simulink model "pv_storage_system"  (R2026a)
settings: Solver=ode23tb
values from neighbouring files (symbols this model uses):
  Batt_AhRated = 100    [pv_storage_params.m]
  f_sw_bb = 8e3    (= 8000)    [pv_storage_params.m]
  f_sw_boost = 8e3    (= 8000)    [pv_storage_params.m]
  R1_boost = 0.01    [pv_storage_params.m]
  R_snubber = 2.7    [pv_storage_params.m]
  R_test_load = 480^2 / 30000    (= 7.68)    [pv_storage_params.m]
  R_test_load_batt = 500    [pv_storage_params.m]
  Ts_control = 150e-6    (= 0.00015)    [pv_storage_params.m]
libraries: fl_lib x19, nesl_utility x9, ee_lib x4, ee_lib_for_power_systems x3, simulink x3, batteryecm_lib x1, slpidlib x1
settings Model: Creator=inspiredkhalid  LastModifiedBy=inspiredkhalid

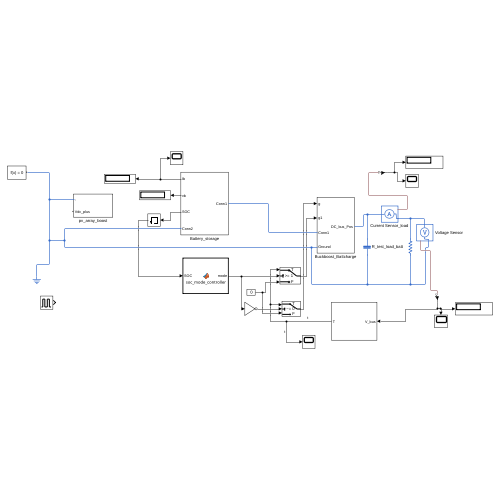
[thumbnail: Simulink's stored preview of the top-level diagram]
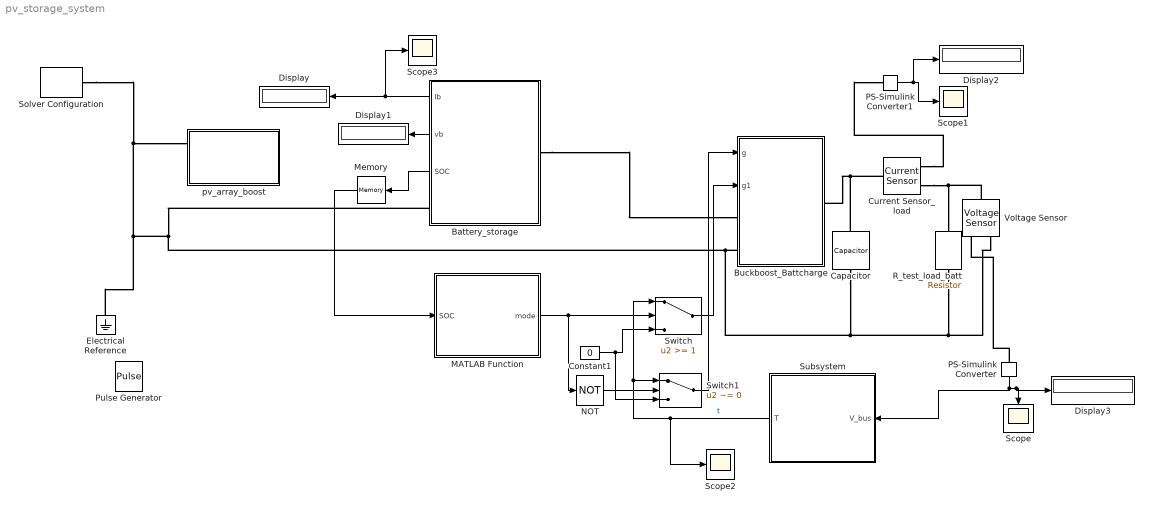
== system pv_storage_system ==
  Battery_storage : Subsystem
  Buckboost_Battcharge : Subsystem
  Capacitor : fl_lib/Electrical/Electrical Elements/Capacitor  c=Cdc F  r=1e-6 Ohm  g=0 1/Ohm  i_specify=off  i_priority=None  i=0 A  i_nominal_specify=off  i_nominal_value=1  i_nominal_unit=A  v_specify=off  v_priority=None  v=0 V  v_nominal_specify=off  v_nominal_value=1  v_nominal_unit=V  vc_specify=off  vc_priority=High  vc=0 V  vc_nominal_specify=off  vc_nominal_value=1  vc_nominal_unit=V
  Constant1 : Constant  Value=0
  Current Sensor_load : fl_lib/Electrical/Electrical Sensors/Current Sensor
  Display{,1..3} (4 alike) : Display
  Electrical Reference : fl_lib/Electrical/Electrical Elements/Electrical Reference
  MATLAB Function : MATLAB Function  TreatAsAtomicUnit=on
  Memory : Memory
  NOT : Logic  Operator=NOT  IconShape=distinctive  AllPortsSameDT=off  OutDataTypeStr=boolean
  PS-Simulink Converter : nesl_utility/PS-Simulink Converter  PhysicalDomain=network_engine_domain  SubClassName=ps_output  LeftPortType=input  RightPortType=output  PseudoPeriodic=off  Frequencies=[]  VectorFormat=inherit  Unit=inherit  AffineConversion=off
  PS-Simulink Converter1 : nesl_utility/PS-Simulink Converter  PhysicalDomain=network_engine_domain  SubClassName=ps_output  LeftPortType=input  RightPortType=output  PseudoPeriodic=off  Frequencies=[]  VectorFormat=inherit  Unit=inherit  AffineConversion=off
  Pulse Generator : DiscretePulseGenerator  PulseType=Time based  Period=1/f_sw_bb  PulseWidth=5
  R_test_load_batt : fl_lib/Electrical/Electrical Elements/Resistor  R=R_test_load_batt Ohm  i_specify=off  i_priority=None  i=0 A  i_nominal_specify=off  i_nominal_value=1  i_nominal_unit=A  v_specify=off  v_priority=None  v=0 V  v_nominal_specify=off  v_nominal_value=1  v_nominal_unit=V
  Scope{,1..3} (4 alike) : Scope
      Scope settings: ActiveDisplayYMinimum=-510.77769359361685  ActiveDisplayYMaximum=637.473510774474  DataLoggingVariableName=ScopeData5
      Scope1 settings: DataLoggingVariableName=ScopeData6
      Scope2 settings: ActiveDisplayYMinimum=0.44778568340914426  ActiveDisplayYMaximum=0.45061540552074841  DataLoggingVariableName=ScopeData7
      Scope3 settings: DataLoggingVariableName=ScopeData9
  Solver Configuration : nesl_utility/Solver Configuration  PhysicalDomain=network_engine_domain  SubClassName=solver  LeftPortType=input  RightPortType=generic  Tones=[]  Harmonics=[]  SimulateNoise=off  Profile=off  UseLocalSampling=off  EnableSwitchedLinearOptims=on  FrequencyDomain=off  UseCCode=off  RelTol=0.001  AbsTol=0.001  MinStep=1e-09  ToWorkspace=off  RevertToSquareIcSolve=off  NumHomotopyIterations=100  PhasorMode=off  PhasorModeNumHarmonics=1  ConsistencySolver=NEWTON_XTOL_AFTER_FTOL  CanonicalOrdering=CANONICAL  OptimizeIntermediates=OPTIMIZED  IndexReductionMethod=DerivativeReplacement  DoDC=off  ResidualTolerance=1e-09  ConsistencyTolSource=GLOBAL  ConsistencyAbsTol=0.001  ConsistencyRelTol=0.001  ConsistencyTolFactor=0.001  UseLocalSolver=on  LocalSolverChoice=NE_TRAPEZOIDAL_ADVANCER  ResolveIndetEquations=on  FunctionEvalNumThread=1  LocalSolverSampleTime=Ts_power  DoFixedCost=off  MaxNonlinIter=3  MaxModeIter=2  ComputeImpulses=off  ImpulseIterations=2  LinearAlgebra=auto  LinearAlgebraNumThread=0  EquationFormulation=NE_TIME_EF  DelaysMemoryBudget=1024  AutomaticFiltering=on  FilteringTimeConstant=0.001  PartitionStorageMethod=AS_NEEDED  PartitionMemoryBudget=1024  PartitionMethod=ROBUST  MultibodyUseLocalSolver=off  MultibodyLocalSolverChoice=ODE1  MultibodyLocalSolverSampleTime=0.001
  Subsystem : Subsystem
  Switch : Switch  Threshold=1  SaturateOnIntegerOverflow=off  InputSameDT=off
  Switch1 : Switch  Criteria=u2 ~= 0  Threshold=1  SaturateOnIntegerOverflow=off  InputSameDT=off
  "Voltage Sensor " : fl_lib/Electrical/Electrical Sensors/Voltage Sensor
  pv_array_boost : Subsystem
  wires:
  Battery_storage/1(Ib) -> Scope3/1, Display/1
  Battery_storage/2(vb) -> Display1/1
  MATLAB Function/1(mode) -> NOT/1, Switch/2
  Subsystem/1(T) -> Scope2/1, Switch/1, Switch1/1  "t"
  Constant1/1 -> Switch1/3, Switch/3
  NOT/1 -> Switch1/2
  Battery_storage/3(SOC) -> Memory/1
  Memory/1 -> MATLAB Function/1(SOC)
  PS-Simulink Converter/1 -> Display3/1, Scope/1, Subsystem/1(V_bus)
  PS-Simulink Converter1/1 -> Display2/1, Scope1/1
  Switch/1 -> Buckboost_Battcharge/2(g1)
  Switch1/1 -> Buckboost_Battcharge/1(g)
  connections:
  Battery_storage/RConn1 -- "Voltage Sensor "/RConn2 -- R_test_load_batt/RConn1 -- Capacitor/RConn1 -- Buckboost_Battcharge/LConn2 -- Electrical Reference/LConn1 -- Solver Configuration/RConn1 -- pv_array_boost/LConn1
  Battery_storage/LConn1 -- Buckboost_Battcharge/LConn1
  "Voltage Sensor "/LConn1 -- Current Sensor_load/RConn2 -- R_test_load_batt/LConn1
  PS-Simulink Converter/LConn1 -- "Voltage Sensor "/RConn1
  Current Sensor_load/LConn1 -- Capacitor/LConn1 -- Buckboost_Battcharge/RConn1
  Current Sensor_load/RConn1 -- PS-Simulink Converter1/LConn1

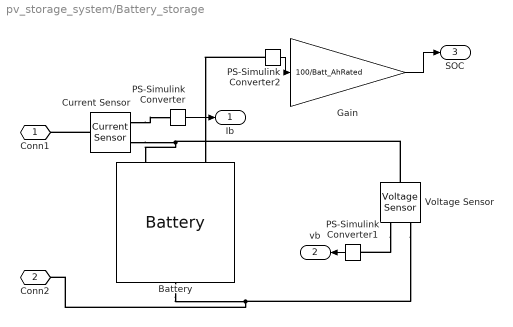
== system pv_storage_system/Battery_storage ==
  Battery : batteryecm_lib/Battery  Vnom=Batt_Vnom V  prm_dir=simscape.enum.battery.prm_dir.disabled  R1_dis=2 Ohm  R1_ch=2 Ohm  R1=Batt_Rint Ohm  prm_AH=simscape.enum.battery.prm_AH.finite  AH=Batt_AhRated A*hr  V1=Batt_V1_calib V  AH1=Batt_AH1_calib A*hr  prm_R2=simscape.enum.battery.prm_R2.disabled  R2=2000 Ohm  Tmeas=298.15 K  charge_measurement_port=simscape.enum.battery.enable.yes  prm_dyn=simscape.enum.battery.prm_dyn.off  Rp1=0.005 Ohm  tau1=30 s  Rp2=0.005 Ohm  tau2=30 s  Rp3=0.005 Ohm  tau3=30 s  Rp4=0.005 Ohm  tau4=30 s  Rp5=0.005 Ohm  tau5=30 s  prm_fade=simscape.enum.battery.prm_fade.disabled  N_fade=100  AH_fade=45 A*hr  R1_fade=2.02 Ohm  R1_ch_fade=2.02 Ohm  V1_fade=10.35 V  prm_age=simscape.enum.battery.prm_age.disabled  prm_age_OCV=simscape.enum.battery.prm_age_OCV.OCV  OCV_age=0.9  SOC_age=60  Tmeas_age=298.15 K  delta_time_age_vec=[0] d  temperature_age_vec=[273] K  OCV_scaling_age=2.2134e6  OCV_offset_age=1.632e6  temp_exp_age=0.515833569 V  t_exp_age=0.75  Vnom_T2=12 V  R1_T2=2.2 Ohm  R1_T2_dis=2.2 Ohm  R1_T2_ch=2.2 Ohm  V1_T2=11.4 V  R2_T2=2200 Ohm  Rp1_T2=0.005 Ohm  tau1_T2=30 s  Rp2_T2=0.005 Ohm  tau2_T2=30 s  Rp3_T2=0.005 Ohm  tau3_T2=30 s  Rp4_T2=0.005 Ohm  tau4_T2=30 s  Rp5_T2=0.005 Ohm  tau5_T2=30 s  Tmeas2=273.15 K  thermal_port=simscape.enum.thermaleffects.omit  thermal_mass=30000 J/K  i_specify=off  i_priority=None  i=0 A  i_nominal_specify=off  i_nominal_value=1  i_nominal_unit=A  v_specify=off  v_priority=None  v=0 V  v_nominal_specify=off  v_nominal_value=1  v_nominal_unit=V  charge_specify=on  charge_priority=High  charge=Batt_Charge_init A*hr  charge_nominal_specify=off  charge_nominal_value=1  charge_nominal_unit=A*hr  num_cycles_specify=off  num_cycles_priority=High  num_cycles=0  num_cycles_nominal_specify=off  num_cycles_nominal_value=1  num_cycles_nominal_unit=1  temperature_specify=off  temperature_priority=High  temperature=298.15 K  temperature_nominal_specify=off  temperature_nominal_value=1  temperature_nominal_unit=K
  Current Sensor : fl_lib/Electrical/Electrical Sensors/Current Sensor
  Gain : Gain  Gain=100/Batt_AhRated
  PS-Simulink Converter : nesl_utility/PS-Simulink Converter  PhysicalDomain=network_engine_domain  SubClassName=ps_output  LeftPortType=input  RightPortType=output  PseudoPeriodic=off  Frequencies=[]  VectorFormat=inherit  Unit=inherit  AffineConversion=off
  PS-Simulink Converter1 : nesl_utility/PS-Simulink Converter  PhysicalDomain=network_engine_domain  SubClassName=ps_output  LeftPortType=input  RightPortType=output  PseudoPeriodic=off  Frequencies=[]  VectorFormat=inherit  Unit=inherit  AffineConversion=off
  PS-Simulink Converter2 : nesl_utility/PS-Simulink Converter  PhysicalDomain=network_engine_domain  SubClassName=ps_output  LeftPortType=input  RightPortType=output  PseudoPeriodic=off  Frequencies=[]  VectorFormat=inherit  Unit=inherit  AffineConversion=off
  Voltage Sensor : fl_lib/Electrical/Electrical Sensors/Voltage Sensor
  Conn1 : PMIOPort  Side=Left
  Conn2 : PMIOPort  Port=2  Side=Right
  Ib : Outport
  vb : Outport  Port=2
  SOC : Outport  Port=3
  wires:
  PS-Simulink Converter/1 -> Ib/1
  PS-Simulink Converter1/1 -> vb/1
  PS-Simulink Converter2/1 -> Gain/1
  Gain/1 -> SOC/1
  connections:
  Battery/RConn1 -- Voltage Sensor/RConn2 -- Conn2/RConn1
  Current Sensor/LConn1 -- Conn1/RConn1
  Voltage Sensor/LConn1 -- Current Sensor/RConn2 -- Battery/LConn1
  Current Sensor/RConn1 -- PS-Simulink Converter/LConn1
  Voltage Sensor/RConn1 -- PS-Simulink Converter1/LConn1
  PS-Simulink Converter2/LConn1 -- Battery/LConn2

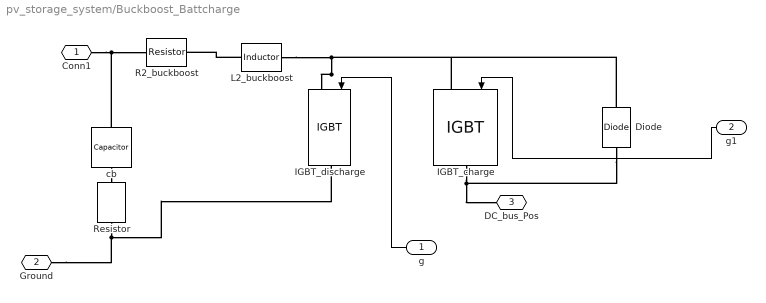
== system pv_storage_system/Buckboost_Battcharge ==
  g : Inport
  g1 : Inport  Port=2
  " IGBT_charge" : ee_lib_for_power_systems/Power Converters/IGBT  Vf=0.6  Ron=1e-3  Goff=1e-5  run_time=off
      settings: SourceProductName=Support Library for Power Systems
  Diode : fl_lib/Electrical/Electrical Elements/Diode  Vf=0.6 V  Ron=0.3 Ohm  Goff=1e-8 1/Ohm  i_specify=off  i_priority=None  i=0 A  i_nominal_specify=off  i_nominal_value=1  i_nominal_unit=A  v_specify=off  v_priority=None  v=0 V  v_nominal_specify=off  v_nominal_value=1  v_nominal_unit=V
  IGBT_discharge : ee_lib_for_power_systems/Power Converters/IGBT  Vf=0.6  Ron=1e-3  Goff=1e-5  run_time=off
      settings: SourceProductName=Support Library for Power Systems
  L2_buckboost : ee_lib/Passive/Inductor  l=1e-6 H  enable_L_tol=ee.enum.toleranceApplication.none  L_tol=20  tol_distribution=ee.enum.toleranceDistribution.uniform  nSigma=4  r=0 Ohm  g=1e-9 1/Ohm  enable_operating_limits=ee.enum.enable.no  operating_limit_action=ee.enum.passive.reportOpLim.warn  max_working_current=1 A  power_rating=1 W  i_L_specify=off  i_L_priority=High  i_L=0 A  i_L_nominal_specify=off  i_L_nominal_value=1  i_L_nominal_unit=A
  R2_buckboost : fl_lib/Electrical/Electrical Elements/Resistor  R=1 Ohm  i_specify=off  i_priority=None  i=0 A  i_nominal_specify=off  i_nominal_value=1  i_nominal_unit=A  v_specify=off  v_priority=None  v=0 V  v_nominal_specify=off  v_nominal_value=1  v_nominal_unit=V
  Resistor : fl_lib/Electrical/Electrical Elements/Resistor  R=R_snubber Ohm  i_specify=off  i_priority=None  i=0 A  i_nominal_specify=off  i_nominal_value=1  i_nominal_unit=A  v_specify=off  v_priority=None  v=0 V  v_nominal_specify=off  v_nominal_value=1  v_nominal_unit=V
  cb : fl_lib/Electrical/Electrical Elements/Capacitor  c=1e-6 F  r=1e-6 Ohm  g=0 1/Ohm  i_specify=off  i_priority=None  i=0 A  i_nominal_specify=off  i_nominal_value=1  i_nominal_unit=A  v_specify=off  v_priority=None  v=0 V  v_nominal_specify=off  v_nominal_value=1  v_nominal_unit=V  vc_specify=off  vc_priority=High  vc=0 V  vc_nominal_specify=off  vc_nominal_value=1  vc_nominal_unit=V
  Conn1 : PMIOPort  Side=Left
  Ground : PMIOPort  Port=2  Side=Left
  DC_bus_Pos : PMIOPort  Port=3  Side=Right
  wires:
  g/1 -> IGBT_discharge/1
  g1/1 -> " IGBT_charge"/1
  connections:
  " IGBT_charge"/RConn1 -- DC_bus_Pos/RConn1 -- Diode/RConn1
  IGBT_discharge/LConn1 -- Diode/LConn1 -- " IGBT_charge"/LConn1 -- L2_buckboost/RConn1
  cb/LConn1 -- R2_buckboost/LConn1 -- Conn1/RConn1
  L2_buckboost/LConn1 -- R2_buckboost/RConn1
  Ground/RConn1 -- IGBT_discharge/RConn1 -- Resistor/RConn1
  cb/RConn1 -- Resistor/LConn1

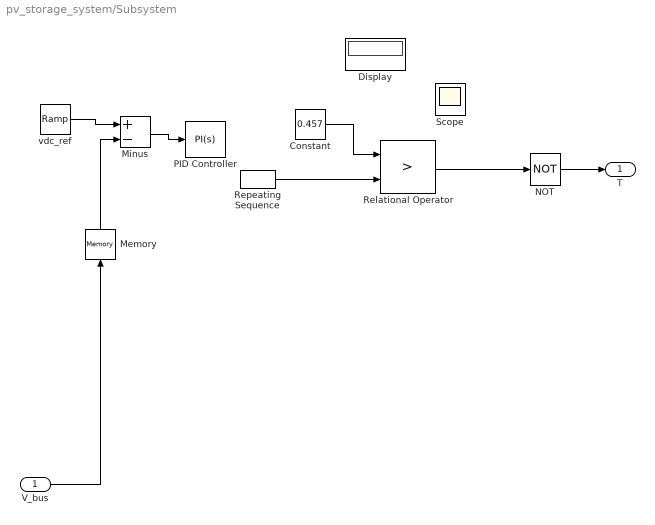
== system pv_storage_system/Subsystem ==
  V_bus : Inport
  Constant : Constant  Value=0.457
  Display : Display
  Memory : Memory
  Minus : Sum  Inputs=+-
  NOT : Logic  Operator=NOT  IconShape=distinctive  AllPortsSameDT=off  OutDataTypeStr=boolean
  PID Controller : slpidlib/PID Controller  Controller=PI  Form=Parallel  TimeDomain=Continuous-time  UseExternalTs=off  SampleTime=-1  IntegratorMethod=Forward Euler  FilterMethod=Forward Euler  ControllerParametersSource=internal  P=0.001  I=0.1  UseKiTs=off  D=0  UseExternalDerivativeSource=off  N=100  UseFilter=on  TunerSelectOption=Transfer Function Based (PID Tuner App)  InitialConditionSource=internal  InitialConditionForIntegrator=0  InitialConditionForFilter=0  DifferentiatorICPrevScaledInput=0  ExternalReset=none  TrackingMode=off  Kt=1  LimitOutput=on  SatLimitsSource=internal  UpperSaturationLimit=0.85  LowerSaturationLimit=0  LinearizeAsGain=on  AntiWindupMode=clamping  Kb=1  LimitIntegrator=off  UpperIntegratorSaturationLimit=inf  LowerIntegratorSaturationLimit=-inf  POutMin=[]  POutMax=[]  IOutMin=[]  IOutMax=[]  DOutMin=[]  DOutMax=[]  NOutMin=[]  NOutMax=[]  SumOutMin=[]  SumOutMax=[]  SaturationOutMin=[]  SaturationOutMax=[]  PParamMin=[]  PParamMax=[]  IParamMin=[]  IParamMax=[]  DParamMin=[]  DParamMax=[]  NParamMin=[]  NParamMax=[]  KbParamMin=[]  KbParamMax=[]  KtParamMin=[]  KtParamMax=[]  KbOutMin=[]  KbOutMax=[]  KtOutMin=[]  KtOutMax=[]  IntegratorOutMin=[]  IntegratorOutMax=[]  FilterOutMin=[]  FilterOutMax=[]  SumI1OutMin=[]  SumI1OutMax=[]  SumI2OutMin=[]  SumI2OutMax=[]  SumI3OutMin=[]  SumI3OutMax=[]  SumI4OutMin=[]  SumI4OutMax=[]  SumDOutMin=[]  SumDOutMax=[]  DifferentiatorOutMin=[]  DifferentiatorOutMax=[]  FilterDiffOutCoefMin=[]  FilterDiffOutCoefMax=[]  ReciprocalOutMin=[]  ReciprocalOutMax=[]  SumDenOutMin=[]  SumDenOutMax=[]  SumNumOutMin=[]  SumNumOutMax=[]  DivideOutMin=[]  DivideOutMax=[]  UdiffTsProdOutMin=[]  UdiffTsProdOutMax=[]  NTsProdOutMin=[]  NTsProdOutMax=[]  UintegralTsProdOutMin=[]  UintegralTsProdOutMax=[]  UngainTsProdOutMin=[]  UngainTsProdOutMax=[]  ClampingZeroOutDataTypeStr=Inherit: Inherit via back propagation  ClampingZeroOutMin=[]  ClampingZeroOutMax=[]  FilterDenConstantOutDataTypeStr=Inherit: Inherit via back propagation  FilterDenConstantOutMin=[]  FilterDenConstantOutMax=[]  PCopyOutDataTypeStr=Inherit: Inherit via back propagation  PCopyOutMin=[]  PCopyOutMax=[]  NCopyOutDataTypeStr=Inherit: Inherit via back propagation  NCopyOutMin=[]  NCopyOutMax=[]  IntegratorContinuousStateAttributes=''  IntegratorStateMustResolveToSignalObject=off  IntegratorRTWStateStorageClass=Auto  FilterContinuousStateAttributes=''  FilterStateMustResolveToSignalObject=off  FilterRTWStateStorageClass=Auto  ParallelPVariant=InternalParameters  IdealPVariant=Disabled  IVariant=InternalParameters  DVariant=Disabled  IntegratorVariant=Continuous  SatVariant=Enabled  AWVariant=ContClampingParallel  PCopyVariant=Disabled  TRVariant=Disabled  FdbkBlocksVariant=Forward  IdealPFdbkVariant=Disabled  SatFdbkVariant=Disabled  DerivativeFilterVariant=Disabled  NVariant=Disabled  NCopyVariant=Disabled_SignalSpec  FilterICVariant=Disabled  IntegratorICVariant=InternalICs  ExternalResetVariant=Disabled  TRSumVariant=Passthrough  SumFdbkVariant=Disabled  SumVariant=Sum_PI  TsampFilterVariant=InternalTs  TsampNgainVariant=Passthrough  TsampIntegralVariant=Disabled_SignalSpec  ExternalSaturationOutDataTypeStr=Inherit: Same as second input  DerivativeSourceVariant=Disabled  PreIntVariant=InternalPreInt
  Relational Operator : RelationalOperator  Operator=>  OutDataTypeStr=boolean  RndMeth=Simplest  InputSameDT=off
  Repeating Sequence : simulink/Sources/Repeating Sequence  rep_seq_t=[0 1/f_sw_bb]  rep_seq_y=[0 1]
  Scope : Scope
      settings: ActiveDisplayYMinimum=0.96541730097571365  ActiveDisplayYMaximum=1.0189869647757612  DataLoggingVariableName=ScopeData8
  vdc_ref : simulink/Sources/Ramp  slope=500  start=0  InitialOutput=0
  T : Outport
  wires:
  Repeating Sequence/1 -> Relational Operator/2
  Minus/1 -> PID Controller/1
  vdc_ref/1 -> Minus/1
  V_bus/1 -> Memory/1
  Memory/1 -> Minus/2
  NOT/1 -> T/1
  Relational Operator/1 -> NOT/1
  Constant/1 -> Relational Operator/1

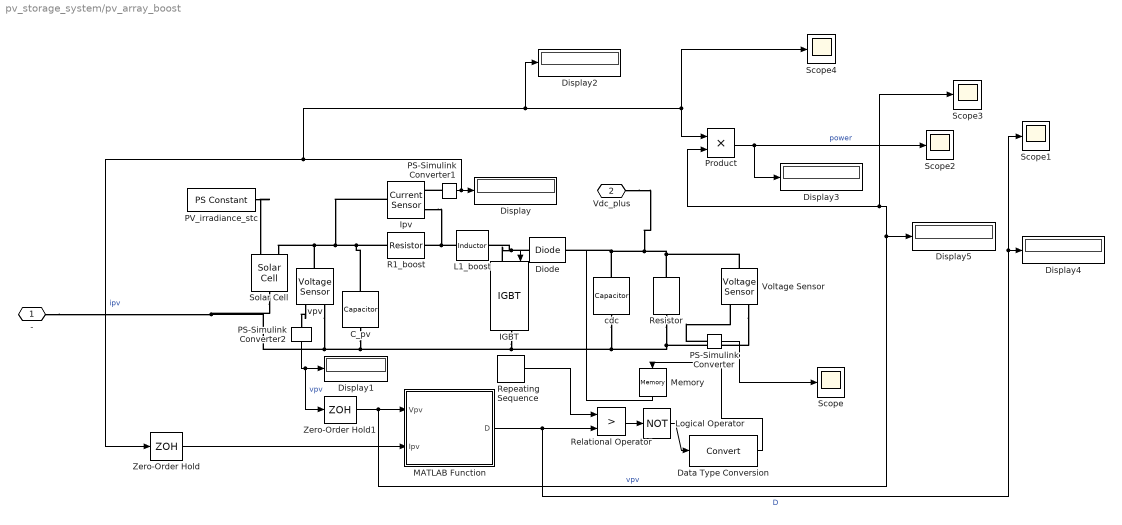
== system pv_storage_system/pv_array_boost ==
  C_pv : fl_lib/Electrical/Electrical Elements/Capacitor  c=C_pv F  r=1e-6 Ohm  g=0 1/Ohm  i_specify=off  i_priority=None  i=0 A  i_nominal_specify=off  i_nominal_value=1  i_nominal_unit=A  v_specify=off  v_priority=None  v=0 V  v_nominal_specify=off  v_nominal_value=1  v_nominal_unit=V  vc_specify=off  vc_priority=High  vc=0 V  vc_nominal_specify=off  vc_nominal_value=1  vc_nominal_unit=V
  Data Type Conversion : DataTypeConversion  SaturateOnIntegerOverflow=off  RndMeth=Floor
  "Diode " : ee_lib/Semiconductors & Converters/Diode  ModelType=ee.enum.diode.modelType.pwl  TableType=ee.enum.diode.tableType.IfMat  IfMat=[.07, .12, .19, 1.75, 4.24, 7.32, 11.2; .16, .3, .72, 2.14, 5.02, 8.35, 13.12] A  VfMat=[.9, 1.15, 1.25, 1.5, 1.75, 2.17, 2.6, 2.85; .58, .68, .75, 1.1, 1.38, 1.77, 2.27, 2.7] V  TjVec=[25, 125] degC  VfVec=[.5, .7, .9, 1.3, 1.7, 2.1, 2.5] V  IfVec=[.1, .2, .5, 1, 2, 4, 7, 10] A  IrMat=[1e-06, 2e-06, 5e-06, 1e-05, 2.5e-05, 5e-05, .0001; 2e-06, 5e-06, 1e-05, 4e-05, 8e-05, .0002, .0005] A  VrMat=[10, 100, 200, 250, 300, 325, 350; 10, 70, 160, 220, 270, 300, 320] V  VrVec=[10, 20, 40, 50, 70, 80, 100] V  IrVec=[1e-06, 2e-06, 5e-06, 1e-05, 2e-05, 5e-05, .0001] A  Vf=0.6 V  Ron=0.3 Ohm  Goff=1e-8 S  prmExp=ee.enum.diode.expParam.useTwo  I12=[.0137, .545] A  V12=[.6, .7] V  RS=0 Ohm  Tmeas=298.15 K  IS=1e-12 A  ec=1  I1=0.0137 A  V1=0.6 V  N_series=1  N_parallel=1  ZenerEnable=false  Rz=0.3 Ohm  BV=30 V  C_param=ee.enum.diode.capParam.fixed  CJ=0 pF  CJ0=5 pF  Vvec=[.1, 10, 100] V  Cvec=[3.5, 1, .4] pF  VJ=1 V  Mgrad=0.5  FC=0.5  Q_param=ee.enum.diode.recoveryParam.off  iRM=-7.15 A  iF=4 A  didt=-750 A/us  trr_factor=3  trr=115 ns  Qrr=150 nA*s  Vr=-600 V  Ls=150 nH  Erec=0.03 J  TT=50 ns  tau=100 ns  T_param=ee.enum.diode.temperatureParam.off  Tdevice=298.15 K  I1_T2=0.245 A  V1_T2=0.5 V  IS_T2=1.25e-7 A  Tmeas2=125 degC  XTI_param=ee.enum.diode.xtiParam.pn  XTI=3  EG_param=ee.enum.diode.egapParam.material_si  EG=1.11 eV  dBVdT=0 V/K  enable_fault_input=simscape.enum.onoff.off  i_specify=off  i_priority=None  i=0 A  i_nominal_specify=off  i_nominal_value=1  i_nominal_unit=A  v_specify=off  v_priority=None  v=0 V  v_nominal_specify=off  v_nominal_value=1  v_nominal_unit=V  v_capacitor_specify=off  v_capacitor_priority=None  v_capacitor=0 V  v_capacitor_nominal_specify=off  v_capacitor_nominal_value=1  v_capacitor_nominal_unit=V  Qj_specify=off  Qj_priority=High  Qj=0 C  Qj_nominal_specify=off  Qj_nominal_value=1  Qj_nominal_unit=C  i_diode_specify=off  i_diode_priority=None  i_diode=0 A  i_diode_nominal_specify=off  i_diode_nominal_value=1  i_diode_nominal_unit=A  v_diode_specify=off  v_diode_priority=None  v_diode=0 V  v_diode_nominal_specify=off  v_diode_nominal_value=1  v_diode_nominal_unit=V  i_capacitor_specify=off  i_capacitor_priority=None  i_capacitor=0 A  i_capacitor_nominal_specify=off  i_capacitor_nominal_value=1  i_capacitor_nominal_unit=A  fidelity_level=ee.enum.diode.fidelity.includeChargeDyn  rec_loss_model=ee.enum.diode.reverseRecoveryModelTabulateUpTo3D.fixed  ErecVal=0 J  scaleWithIandV=true  ErecMat=zeros(2, 3) J  ErecMat3D=zeros(2, 3, 2) J  TjrecVec=[298.15, 398.15] K  IfrecVec=[.1, 1, 10] A  IrecVal=10 A  VrecVal=10 V  VrecVec=[0, 100] V  tFilter=1 / 1000 / 100 s  thermal_network_parameterization=ee.enum.thermalNetworkTopology.junctionCase  Rth=[0, 10] K/W  Rth_Cauer=[1, 3, 10] K/W  Rth_Foster=[.08, .14, .22, .16] K/W  thermal_mass_parameterization=ee.enum.thermalNetwork.timeconstant  thermal_mass=[0, 1] J/K  thermal_mass_Cauer=[.1, .3, 1] J/K  thermal_mass_Foster=[.001, .005, .05, .5] J/K  thermal_time_constant=[0, 10] s  thermal_time_constant_Cauer=[1, 3, 10] s  thermal_time_constant_Foster=[7e-05, .0007, .01, .08] s  thermal_mass_initial_temperatures=[25, 25] degC  thermal_mass_initial_temperatures_Cauer=[25, 25, 25] degC  junction_thermal_mass=0.01 J/K  Tvec_initial_Foster=[25, 25, 25, 25] degC  no_thermal_network=0  junction_temperature_specify=off  junction_temperature_priority=None  junction_temperature=25 degC  junction_temperature_nominal_specify=off  junction_temperature_nominal_value=1  junction_temperature_nominal_unit=degC
  Display{,1..5} (6 alike) : Display
  IGBT : ee_lib_for_power_systems/Power Converters/IGBT  Vf=0.6  Ron=1e-3  Goff=1e-5  run_time=off
      settings: SourceProductName=Support Library for Power Systems
  Ipv : fl_lib/Electrical/Electrical Sensors/Current Sensor
  L1_boost : ee_lib/Passive/Inductor  l=L1_boost H  enable_L_tol=ee.enum.toleranceApplication.none  L_tol=20  tol_distribution=ee.enum.toleranceDistribution.uniform  nSigma=4  r=0 Ohm  g=1e-9 1/Ohm  enable_operating_limits=ee.enum.enable.no  operating_limit_action=ee.enum.passive.reportOpLim.warn  max_working_current=1 A  power_rating=1 W  i_L_specify=off  i_L_priority=High  i_L=0 A  i_L_nominal_specify=off  i_L_nominal_value=1  i_L_nominal_unit=A
  Logical Operator : Logic  Operator=NOT  AllPortsSameDT=off  OutDataTypeStr=boolean
  MATLAB Function : MATLAB Function  TreatAsAtomicUnit=on
  Memory : Memory
  PS-Simulink Converter : nesl_utility/PS-Simulink Converter  PhysicalDomain=network_engine_domain  SubClassName=ps_output  LeftPortType=input  RightPortType=output  PseudoPeriodic=off  Frequencies=[]  VectorFormat=inherit  Unit=inherit  AffineConversion=off
  PS-Simulink Converter1 : nesl_utility/PS-Simulink Converter  PhysicalDomain=network_engine_domain  SubClassName=ps_output  LeftPortType=input  RightPortType=output  PseudoPeriodic=off  Frequencies=[]  VectorFormat=inherit  Unit=inherit  AffineConversion=off
  PS-Simulink Converter2 : nesl_utility/PS-Simulink Converter  PhysicalDomain=network_engine_domain  SubClassName=ps_output  LeftPortType=input  RightPortType=output  PseudoPeriodic=off  Frequencies=[]  VectorFormat=inherit  Unit=inherit  AffineConversion=off
  PV_irradiance_stc : fl_lib/Physical Signals/Sources/PS Constant  constant=PV_irradiance_STC
  Product : Product
  R1_boost : fl_lib/Electrical/Electrical Elements/Resistor  R=R1_boost Ohm  i_specify=off  i_priority=None  i=0 A  i_nominal_specify=off  i_nominal_value=1  i_nominal_unit=A  v_specify=off  v_priority=None  v=0 V  v_nominal_specify=off  v_nominal_value=1  v_nominal_unit=V
  Relational Operator : RelationalOperator  Operator=>  OutDataTypeStr=boolean  RndMeth=Simplest  InputSameDT=off
  Repeating Sequence : simulink/Sources/Repeating Sequence  rep_seq_t=[0 1/f_sw_boost]  rep_seq_y=[0 1]
  Resistor : fl_lib/Electrical/Electrical Elements/Resistor  R=R_test_load Ohm  i_specify=off  i_priority=None  i=0 A  i_nominal_specify=off  i_nominal_value=1  i_nominal_unit=A  v_specify=off  v_priority=None  v=0 V  v_nominal_specify=off  v_nominal_value=1  v_nominal_unit=V
  Scope{,1..4} (5 alike) : Scope
      Scope settings: ActiveDisplayYMinimum=-1419.4876054111123  ActiveDisplayYMaximum=2958.224359813305
      Scope1 settings: ActiveDisplayYMinimum=0.36784943892587946  ActiveDisplayYMaximum=0.41398203833502917
      Scope2 settings: ActiveDisplayYMinimum=-1  ActiveDisplayYMaximum=1  DataLoggingVariableName=ScopeData2
      Scope3 settings: ActiveDisplayYMinimum=-689.02233438403414  ActiveDisplayYMaximum=763.06983633368964  DataLoggingVariableName=ScopeData3
      Scope4 settings: ActiveDisplayYMinimum=-39.0838718758448  ActiveDisplayYMaximum=351.75484688260559  DataLoggingVariableName=ScopeData4
  "Solar Cell " : ee_lib/Sources/Solar Cell  prm=ee.enum.sources.solar_cell_prm.datasheet  Isc=7.34 A  Voc=0.6 V  Is=1e-6 A  Is2=0 A  Iph=7.34 A  Ir0=PV_irradiance_STC W/m^2  ec=1.5  N2=2  Rs=0 Ohm  Rp=inf Ohm  N_series=PV_Ns_series_cells  N_parallel=PV_Np_parallel_str  TIPH1=0 1/K  EG=1.11 eV  TXIS1=3  TXIS2=3  TRS1=0  TRP1=0  Tmeas=PV_temp_STC degC  TFIXED=25 degC  thermal_mass=100 J/K  initial_temperature=25 degC
  Voltage Sensor : fl_lib/Electrical/Electrical Sensors/Voltage Sensor
  Zero-Order Hold : ZeroOrderHold  SampleTime=Ts_control
  Zero-Order Hold1 : ZeroOrderHold  SampleTime=Ts_control
  cdc : fl_lib/Electrical/Electrical Elements/Capacitor  c=Cdc F  r=1e-6 Ohm  g=0 1/Ohm  i_specify=off  i_priority=None  i=0 A  i_nominal_specify=off  i_nominal_value=1  i_nominal_unit=A  v_specify=off  v_priority=None  v=0 V  v_nominal_specify=off  v_nominal_value=1  v_nominal_unit=V  vc_specify=off  vc_priority=High  vc=0 V  vc_nominal_specify=off  vc_nominal_value=1  vc_nominal_unit=V
  vpv : fl_lib/Electrical/Electrical Sensors/Voltage Sensor
  - : PMIOPort  Side=Left
  Vdc_plus : PMIOPort  Port=2  Side=Left
  wires:
  Data Type Conversion/1 -> Memory/1
  Zero-Order Hold/1 -> MATLAB Function/2(Ipv)
  PS-Simulink Converter2/1 -> Zero-Order Hold1/1, Display1/1  "vpv"
  PS-Simulink Converter/1 -> Scope/1
  PS-Simulink Converter1/1 -> Display2/1, Scope4/1, Product/1, Zero-Order Hold/1, Display/1  "ipv"
  Repeating Sequence/1 -> Relational Operator/1
  Zero-Order Hold1/1 -> Display5/1, Scope3/1, Product/2, MATLAB Function/1(Vpv)  "vpv"
  Memory/1 -> IGBT/1
  Relational Operator/1 -> Logical Operator/1
  Logical Operator/1 -> Data Type Conversion/1
  MATLAB Function/1(D) -> Scope1/1, Display4/1, Relational Operator/2  "D"
  Product/1 -> Scope2/1, Display3/1  "power"
  connections:
  PV_irradiance_stc/RConn1 -- "Solar Cell "/LConn1
  vpv/RConn1 -- PS-Simulink Converter2/LConn1
  cdc/LConn1 -- Voltage Sensor/LConn1 -- Resistor/LConn1 -- Vdc_plus/RConn1 -- "Diode "/RConn1
  "Solar Cell "/RConn1 -- -/RConn1 -- vpv/RConn2 -- Voltage Sensor/RConn2 -- Resistor/RConn1 -- cdc/RConn1 -- IGBT/RConn1 -- C_pv/RConn1
  PS-Simulink Converter/LConn1 -- Voltage Sensor/RConn1
  R1_boost/LConn1 -- C_pv/LConn1 -- Ipv/LConn1 -- vpv/LConn1 -- "Solar Cell "/LConn2
  PS-Simulink Converter1/LConn1 -- Ipv/RConn1
  "Diode "/LConn1 -- IGBT/LConn1 -- L1_boost/RConn1
  L1_boost/LConn1 -- Ipv/RConn2 -- R1_boost/RConn1

== matlab function pv_storage_system/pv_array_boost/MATLAB Function ==
  data: Vpv input; D output; Ipv input
function D = pv_mppt_po(Vpv, Ipv)
%#codegen
persistent D_prev P_prev V_prev dir_prev
if isempty(D_prev)
    D_prev = 0.5;
    P_prev = 0;
    V_prev = 0;
    dir_prev = 1;
end

dD = 0.005;
D_min = 0.1;
D_max = 0.9;

P = Vpv * Ipv;
dP = P - P_prev;
dV = Vpv - V_prev;

if dP > 0
    if dV > 0
        dir = -1;
    else
        dir = 1;
    end
elseif dP < 0
    if dV > 0
        dir = 1;
    else
        dir = -1;
    end
else
    dir = dir_prev;   % tie: keep perturbing in the same direction, never freeze
end

D = D_prev + dir * dD;
D = min(max(D, D_min), D_max);

D_prev = D;
P_prev = P;
V_prev = Vpv;
dir_prev = dir;
end

== matlab function pv_storage_system/MATLAB Function ==
  data: SOC input; mode output
function mode = soc_mode_controller(SOC)
%#codegen
persistent mode_prev
if isempty(mode_prev)
    mode_prev = 0;   % 0 = discharge, 1 = charge
end

SOC_target = 60;
SOC_hyst = 5;

if SOC < (SOC_target - SOC_hyst)
    mode = 1;    % charge
elseif SOC > (SOC_target + SOC_hyst)
    mode = 0;    % discharge
else
    mode = mode_prev;
end

mode_prev = mode;
end
